simulink model "sin_model"  (R2022a)
settings: Solver=VariableStepAuto  StartTime=0.0  StopTime=10.0  RelTol=1e-3
PreLoadFcn:
  | sin_params
undefined symbols (not defined in the file): A, w
settings Model: Creator=User  LastModifiedBy=DI_Adam
settings DebuggingCC: UnconnectedInputMsg=warning  UnconnectedOutputMsg=warning  UnconnectedLineMsg=warning
settings RTWCC: DLArmComputeVersion=19.05

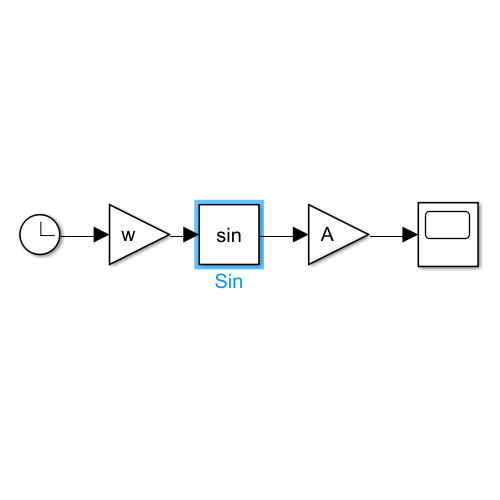
[thumbnail: Simulink's stored preview of the top-level diagram]
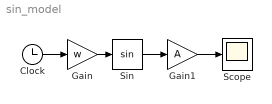
== system sin_model ==
  Clock : Clock
  Gain : Gain  Gain=w
  Gain1 : Gain  Gain=A
  Scope : Scope
  Sin : Trigonometry
  wires:
  Clock/1 -> Gain/1
  Gain/1 -> Sin/1
  Sin/1 -> Gain1/1
  Gain1/1 -> Scope/1
